simulink model "CAVE_MachE_Simulink_250904"  (R2024a)
settings: configuration reference "ConfigSetDesktopFixedStep" (kept outside this file)
PreLoadFcn:
  | VSS_BICYCLE=Simulink.Variant('Dual=0');
  | VSS_DUAL=Simulink.Variant('Dual=1');
  | Dual=1;
  | load('DriveCycle2.mat')
PostLoadFcn:
  | if any(exist('dsrtsu_mdlpostloadfcn', 'file') ~= 0), dsrtsu_mdlpostloadfcn('Execute', bdroot); end
InitFcn:
  | , if any(exist('rtifpga_mdlclblib', 'file') ~= 0), rtifpga_mdlclblib('Init', bdroot); end,
  | , if any(exist('dsmpb_private', 'file') ~= 0), dsmpb_private('dsmpb_mdlclblib', 'Init', bdroot); end,
  | load('DriveCycle2.mat')
model workspace (MAT data in the model file):
  Gas = 0.383333333333
values from neighbouring files (symbols this model uses):
  CoastDown =     [Run_Simulink.mat]
  limitedMCT =     [Run_Simulink.mat]
  MCT =     [Run_Simulink.mat]
  pMCT =     [Run_Simulink.mat]
  RealSimPara =     [Run_Simulink.mat]
  Ref_speed = [13 13.007895099 13.015778396 13.023649891 13.031509584 13.039357475 13.047193564 13.055017851 13.062830336 13.070631019 13.0784199 13.086196979 ... (2669 elements, 2669x1)]    [Ref_speed_and_time.mat]
  Ref_time = [0 0.01 0.02 0.03 0.04 0.05 0.06 0.07 0.08 0.09 0.1 0.11 ... (2669 elements, 2669x1)]    [Ref_speed_and_time.mat]
  US06 =     [Run_Simulink.mat]
undefined symbols (not defined in the file or in its folder): AccelCmd, ActTqLF_Nm_, ActTqLR_Nm_, ActTqRF_Nm_, ActTqRR_Nm_, BattChargeLimitMaxPwr, BattChargeLimitSocBpts, BattChargeLimitTbl, BattChrgCapcty, BattDischargeLimitSocBpts, BattDischargeLimitTbl, BattDischargeMaxPwr, BattNumCellsParallel, BattNumCellsSeries, BattOpenVoltCapBpts, BattOpenVoltTbl, BattResistSocBpts, BattResistTbl, BattResistTempBpts, BrakeMaxPrs, BrakeMaxTrq, ChassisDistCg2FrontAxle, ChassisDistCg2RearAxle, ChassisVehMass, CltchCmd, DecelCmd, DiffRatio, DiscIntNeverNeededParam, EnvGravCnst, EnvPrs, EnvTemp, FuelSpecificGrav, GearCmd, h, InitStates, lgSw, MtrEffSpdBpts, MtrEffTbl, MtrEffTrqBpts, MtrPwrMax, MtrTrqMax, SteeringCmd, SupvsryCtrlRegenBrkCutOffTbl, SupvsryCtrlRegenSpdBpts, TestScnrioCycleNum, VEH
libraries: VSIGenLib x122, simulink x108, etargetslib x75, dsmpblib x41, vehdynlibtire x24, autolibshared x19, vehdynlibsuspension x14, vehdynlibtirecommon x14, autolibutils x10, CarMaker4SL x8, VsrLibWheel x8, autolibpowerinfoutils x6
(part 4 of 29)

== system CAVE_MachE_Simulink_250904/Vehicle Under Test2/Vehicle/Motor ==
  SupvsryCtrl : Inport
  MtrSpd : Inport  Port=2
  Bus Creator1 : BusCreator  Inputs=1
  Bus Creator2 : BusCreator  Inputs=4
  Bus Selector1 : BusSelector  OutputSignals=Volt
  Bus Selector2 : BusSelector  OutputSignals=MtrTrqCmd
  Bus Selector3 : BusSelector  OutputSignals=PwrInfo.PwrTrnsfrd.PwrMtr,PwrInfo.PwrTrnsfrd.PwrBus
  Mach-E Motor : autolibmappedmotor/Mapped Motor  port_config=Speed  param_by=Maximum torque and power  w_t=[ 0 375 750 800 ]  T_t=[0.09 0.08 0.07 0]  torque_max=800  power_max=358000  Tc=0.01  param_loss=Tabulated efficiency data  eff=100  w_eff=375  T_eff=0.08  Piron=0  Pbase=0  w_eff_bp=MtrEffSpdBpts.*pi/30  T_eff_bp=MtrEffTrqBpts  Temp_eff_bp=[233.15 293.15 373.15]  losses_table=[1 2;3 4]  losses_table_3d=cat(3,[1.49 1.67 2.21 3.10; 0.42 0.69 1.14 2.03; 0.06 0.24 0.78 1.68; 0.42 0.69 1.14 2.03; 1.49 1.67 2.21 3.10],[1.49 1.67 2.21 3.10; 0.42 0.69 1.14 2.03; 0.06 0.24 0.78 1.68; 0.42 0.69 1.14 2.03; 1.49 1.67 2.21 3.10],[1.49 1.67 2.21 3.10; 0.42 0.69 1.14 2.03; 0.06 0.24 0.78 1.68; 0.42 0.69 1.14 2.03; 1.49 1.67 2.21 3.10])  efficiency_table=MtrEffTbl*0.94  efficiency_table_3d=cat(3,[95 95 95 95; 95 95 95 95; 95 95 95 95; 95 95 95 95; 95 95 95 95],[95 95 95 95; 95 95 95 95; 95 95 95 95; 95 95 95 95; 95 95 95 95],[95 95 95 95; 95 95 95 95; 95 95 95 95; 95 95 95 95; 95 95 95 95])  J=5e-6  b=1e-5  omega_o=0  T_t_extended=[0 0.07 0.08 0.09 0.08 0.07 0]  w_t_extended=[-800 -750 -375 0 375 750 800]  KLossIron=0  KLossCopper=0  x_w_eff_vec=[-1047.1975511966 -942.477796076938 -837.758040957278 -733.038285837618 -628.318530717959 -523.598775598299 -418.879020478639 -314.159265358979 -285.714285713875 -209.43951023932 -104.71975511966 0 104.71975511966 209.43951023932 285.714285713875 314.159265358979 418.879020478639 523.598775598299 628.318530717959 733.038285837618 837.758040957278 942.477796076938 1047.1975511966]  x_T_eff_vec=[-360 -334.285714285714 -308.571428571429 -282.857142857143 -257.142857142857 -231.428571428571 -205.714285714286 -180 -154.285714285714 -128.571428571429 -102.857142857143 -77.1428571428572 -51.4285714285714 -25.7142857142857 0 25.7142857142857 51.4285714285714 77.1428571428572 102.857142857143 128.571428571429 154.285714285714 180 205.714285714286 231.428571428571 257.142857142857 282.857142857143 308.571428571429 334.285714285714 360]  x_tmp_eff_vec=[-0.09 -0.06 -0.03 0 0.03 0.06 0.09]  x_losses_mat=[54250.1517943165 50375.1409518653 46500.1301094142 42625.119266963 38750.1084245118 34875.0975820605 31000.0867396095 27125.0758971582 23250.065054707 19375.054212256 15500.0433698047 12629.4764797412 9803.55154311708 6774.11181875432 0 5412.5153431847 8293.80460547705 10921.9712596802 13550.1379138833 16937.6723923542 20325.2068708249 23712.7413492957 27100.2758277666 30487.8103062373 33875.3447847082 37262.879263179 40650.4137416499 44037.9482201206 47425.4826985915;44696.230836134 41503.6429192672 38311.0550024006 35118.4670855338 31925.8791686671 28733.2912518003 25540.7033349337 22348.115418067 19155.5275012002 15962.9395843336 12770.3516674669 9577.76375060014 6975.01951641212 6096.70063687888 0 4871.26380886623 6097.56206124747 8462.91205003029 11283.8827333737 14104.8534167172 16925.8241000605 19746.794783404 22567.7654667475 25388.7361500908 28209.7068334343 31030.6775167777 33851.6482001212 36672.6188834645 39493.589566808;36137.1105685043 33555.8883850397 30974.6662015752 28393.4440181105 25812.2218346459 23230.9996511813 20649.7774677168 18068.5552842522 15487.3331007875 12906.110917323 10324.8887338584 8513.56777831124 6200.01734792188 5419.28945500345 0 4330.01227454776 5420.05516555331 7522.58848891581 9220.12563933554 11525.1570491694 13830.1884590033 16135.2198688372 18440.2512786711 20745.2826885049 23050.3140983388 25355.3455081727 27660.3769180066 29965.4083278404 32270.4397376744;31619.9717474413 29361.4023369097 27102.8329263783 24844.2635158467 22585.6941053152 20327.1246947836 18068.5552842522 15809.9858737206 13551.4164631891 11292.8470526576 9034.27764212609 7449.37180602233 5425.01517943165 4741.87827312802 0 3788.76074022929 4742.54826985915 6582.26492780134 8067.6099344186 10084.5124180233 12101.4149016279 14118.3173852325 16135.2198688372 18152.1223524418 20169.0248360465 22185.9273196511 24202.8298032558 26219.7322868604 28236.6347704651;27102.8329263782 25166.9162887798 23230.9996511814 21295.0830135829 19359.1663759844 17423.249738386 15487.3331007876 13551.4164631891 11615.4998255906 9679.58318799226 8513.56777831124 6385.17583373343 4650.01301094141 4064.46709125259 0 3247.50920591082 4065.04137416498 5641.94136668686 7522.58848891582 8643.86778687709 10372.6413442524 12101.4149016279 13830.1884590033 15558.9620163787 17287.7355737541 19016.5091311295 20745.282688505 22474.0562458803 24202.8298032558;22585.6941053152 20972.4302406498 19359.1663759845 17745.9025113191 16132.6386466537 14519.3747819883 12906.110917323 11292.8470526576 9679.58318799221 8066.31932332688 7094.63981525937 5320.97986144452 3875.01084245118 3387.05590937716 0 2706.25767159235 3387.53447847082 4701.61780557238 6268.82374076318 7203.22315573091 8643.86778687704 10084.5124180232 11525.1570491694 12965.8016803156 14406.4463114618 15847.0909426079 17287.7355737541 18728.3802049003 20169.0248360465;19864.9914827262 18446.0635196743 17027.1355566225 15608.2075935706 14189.2796305187 12770.3516674668 11351.423704415 9932.4957413631 8513.56777831121 7094.63981525938 5675.71185220749 4256.78388915562 3100.00867396094 2709.64472750173 0 2165.00613727388 2710.02758277665 3761.29424445791 5015.05899261055 6268.82374076319 7522.58848891579 8776.35323706844 10030.1179852211 11283.8827333737 12537.6474815263 13791.412229679 15045.1769778316 16298.9417259842 17552.7064741369;20587.4582405459 19116.9255090783 17646.3927776108 16175.8600461432 12629.4764797412 11366.528831767 10103.581183793 8137.52276914747 6975.01951641211 5812.51626367679 4650.01301094142 3788.84294392236 2525.89529594824 2032.23354562629 0 1623.75460295541 2184.39425193603 3276.59137790406 4065.04137416499 5081.30171770625 6097.56206124746 7113.82240478872 8737.57700774416 9829.77413371214 10921.9712596802 13684.7775990372 14928.8482898587 16172.9189806802 17416.9896715018;18723.4042552922 17386.0182370571 16048.6322188219 14711.2462005868 11485.9634880614 10337.3671392553 9188.77079044916 8040.174441643 6891.57809283685 5742.98174403074 4594.38539522458 ...(+6536 chars)]  x_losses_mat_3d=[37.8947368421052 25.2631578947368 12.6315789473684 0 12 24 36;18.9473684210526 12.6315789473684 6.3157894736842 0 5.99999999999999 12 18;0 0 0 0 0 0 0;18 12 5.99999999999999 0 6.3157894736842 12.6315789473684 18.9473684210526;36 24 12 0 12.6315789473684 25.2631578947368 37.8947368421052]  CalLossMapData={}  CalLossWithTempMapData={}  aMode=aMode  RefBlkName='autolibmappedmotor/Mapped Motor'
  Mapped Motor : autolibmappedmotor/Mapped Motor  port_config=Speed  param_by=Maximum torque and power  w_t=[ 0 375 750 800 ]  T_t=[0.09 0.08 0.07 0]  torque_max=MtrTrqMax  power_max=MtrPwrMax  Tc=MtrTrqTimeCnst  param_loss=Tabulated efficiency data  eff=100  w_eff=375  T_eff=0.08  Piron=0  Pbase=0  w_eff_bp=MtrEffSpdBpts.*pi/30  T_eff_bp=MtrEffTrqBpts  Temp_eff_bp=[233.15 293.15 373.15]  losses_table=[1 2;3 4]  losses_table_3d=cat(3,[1.49 1.67 2.21 3.10; 0.42 0.69 1.14 2.03; 0.06 0.24 0.78 1.68; 0.42 0.69 1.14 2.03; 1.49 1.67 2.21 3.10],[1.49 1.67 2.21 3.10; 0.42 0.69 1.14 2.03; 0.06 0.24 0.78 1.68; 0.42 0.69 1.14 2.03; 1.49 1.67 2.21 3.10],[1.49 1.67 2.21 3.10; 0.42 0.69 1.14 2.03; 0.06 0.24 0.78 1.68; 0.42 0.69 1.14 2.03; 1.49 1.67 2.21 3.10])  efficiency_table=MtrEffTbl*0.94  efficiency_table_3d=cat(3,[95 95 95 95; 95 95 95 95; 95 95 95 95; 95 95 95 95; 95 95 95 95],[95 95 95 95; 95 95 95 95; 95 95 95 95; 95 95 95 95; 95 95 95 95],[95 95 95 95; 95 95 95 95; 95 95 95 95; 95 95 95 95; 95 95 95 95])  J=5e-6  b=1e-5  omega_o=0  T_t_extended=[0 0.07 0.08 0.09 0.08 0.07 0]  w_t_extended=[-800 -750 -375 0 375 750 800]  KLossIron=0  KLossCopper=0  x_w_eff_vec=[-1047.1975511966 -942.477796076938 -837.758040957278 -733.038285837618 -628.318530717959 -523.598775598299 -418.879020478639 -314.159265358979 -285.714285713875 -209.43951023932 -104.71975511966 0 104.71975511966 209.43951023932 285.714285713875 314.159265358979 418.879020478639 523.598775598299 628.318530717959 733.038285837618 837.758040957278 942.477796076938 1047.1975511966]  x_T_eff_vec=[-360 -334.285714285714 -308.571428571429 -282.857142857143 -257.142857142857 -231.428571428571 -205.714285714286 -180 -154.285714285714 -128.571428571429 -102.857142857143 -77.1428571428572 -51.4285714285714 -25.7142857142857 0 25.7142857142857 51.4285714285714 77.1428571428572 102.857142857143 128.571428571429 154.285714285714 180 205.714285714286 231.428571428571 257.142857142857 282.857142857143 308.571428571429 334.285714285714 360]  x_tmp_eff_vec=[-0.09 -0.06 -0.03 0 0.03 0.06 0.09]  x_losses_mat=[54250.1517943165 50375.1409518653 46500.1301094142 42625.119266963 38750.1084245118 34875.0975820605 31000.0867396095 27125.0758971582 23250.065054707 19375.054212256 15500.0433698047 12629.4764797412 9803.55154311708 6774.11181875432 0 5412.5153431847 8293.80460547705 10921.9712596802 13550.1379138833 16937.6723923542 20325.2068708249 23712.7413492957 27100.2758277666 30487.8103062373 33875.3447847082 37262.879263179 40650.4137416499 44037.9482201206 47425.4826985915;44696.230836134 41503.6429192672 38311.0550024006 35118.4670855338 31925.8791686671 28733.2912518003 25540.7033349337 22348.115418067 19155.5275012002 15962.9395843336 12770.3516674669 9577.76375060014 6975.01951641212 6096.70063687888 0 4871.26380886623 6097.56206124747 8462.91205003029 11283.8827333737 14104.8534167172 16925.8241000605 19746.794783404 22567.7654667475 25388.7361500908 28209.7068334343 31030.6775167777 33851.6482001212 36672.6188834645 39493.589566808;36137.1105685043 33555.8883850397 30974.6662015752 28393.4440181105 25812.2218346459 23230.9996511813 20649.7774677168 18068.5552842522 15487.3331007875 12906.110917323 10324.8887338584 8513.56777831124 6200.01734792188 5419.28945500345 0 4330.01227454776 5420.05516555331 7522.58848891581 9220.12563933554 11525.1570491694 13830.1884590033 16135.2198688372 18440.2512786711 20745.2826885049 23050.3140983388 25355.3455081727 27660.3769180066 29965.4083278404 32270.4397376744;31619.9717474413 29361.4023369097 27102.8329263783 24844.2635158467 22585.6941053152 20327.1246947836 18068.5552842522 15809.9858737206 13551.4164631891 11292.8470526576 9034.27764212609 7449.37180602233 5425.01517943165 4741.87827312802 0 3788.76074022929 4742.54826985915 6582.26492780134 8067.6099344186 10084.5124180233 12101.4149016279 14118.3173852325 16135.2198688372 18152.1223524418 20169.0248360465 22185.9273196511 24202.8298032558 26219.7322868604 28236.6347704651;27102.8329263782 25166.9162887798 23230.9996511814 21295.0830135829 19359.1663759844 17423.249738386 15487.3331007876 13551.4164631891 11615.4998255906 9679.58318799226 8513.56777831124 6385.17583373343 4650.01301094141 4064.46709125259 0 3247.50920591082 4065.04137416498 5641.94136668686 7522.58848891582 8643.86778687709 10372.6413442524 12101.4149016279 13830.1884590033 15558.9620163787 17287.7355737541 19016.5091311295 20745.282688505 22474.0562458803 24202.8298032558;22585.6941053152 20972.4302406498 19359.1663759845 17745.9025113191 16132.6386466537 14519.3747819883 12906.110917323 11292.8470526576 9679.58318799221 8066.31932332688 7094.63981525937 5320.97986144452 3875.01084245118 3387.05590937716 0 2706.25767159235 3387.53447847082 4701.61780557238 6268.82374076318 7203.22315573091 8643.86778687704 10084.5124180232 11525.1570491694 12965.8016803156 14406.4463114618 15847.0909426079 17287.7355737541 18728.3802049003 20169.0248360465;19864.9914827262 18446.0635196743 17027.1355566225 15608.2075935706 14189.2796305187 12770.3516674668 11351.423704415 9932.4957413631 8513.56777831121 7094.63981525938 5675.71185220749 4256.78388915562 3100.00867396094 2709.64472750173 0 2165.00613727388 2710.02758277665 3761.29424445791 5015.05899261055 6268.82374076319 7522.58848891579 8776.35323706844 10030.1179852211 11283.8827333737 12537.6474815263 13791.412229679 15045.1769778316 16298.9417259842 17552.7064741369;20587.4582405459 19116.9255090783 17646.3927776108 16175.8600461432 12629.4764797412 11366.528831767 10103.581183793 8137.52276914747 6975.01951641211 5812.51626367679 4650.01301094142 3788.84294392236 2525.89529594824 2032.23354562629 0 1623.75460295541 2184.39425193603 3276.59137790406 4065.04137416499 5081.30171770625 6097.56206124746 7113.82240478872 8737.57700774416 9829.77413371214 10921.9712596802 13684.7775990372 14928.8482898587 16172.9189806802 17416.9896715018;18723.4042552922 17386.0182370571 16048.6322188219 14711.2462005868 11485.9634880614 10337.3671392553 9188.77079044916 8040.174441643 6891.57809283685 5742.98174403074 4594.38539522458 ...(+6536 chars)]  x_losses_mat_3d=[37.8947368421052 25.2631578947368 12.6315789473684 0 12 24 36;18.9473684210526 12.6315789473684 6.3157894736842 0 5.99999999999999 12 18;0 0 0 0 0 0 0;18 12 5.99999999999999 0 6.3157894736842 12.6315789473684 18.9473684210526;36 24 12 0 12.6315789473684 25.2631578947368 37.8947368421052]  CalLossMapData={}  CalLossWithTempMapData={}  aMode=aMode  RefBlkName='autolibmappedmotor/Mapped Motor'
  Memory : Memory
  Mux{,1..3} (4 alike) : Mux  Inputs=1
  Two-Way Connection1 : TwoWayConnection
  Batt : PMIOPort  Side=Left
  Mtr : Outport
  MtrTrq : Outport  Port=2
  wires:
  Mach-E Motor/3 -> Mux/1, MtrTrq/1  "Trq"
  Mach-E Motor/2 -> Memory/1  "Curr"
  Bus Creator1/1 -> Two-Way Connection1/1
  Mach-E Motor/1 -> Bus Selector3/1
  SupvsryCtrl/1 -> Bus Selector2/1
  Two-Way Connection1/1 -> Bus Selector1/1
  Bus Selector1/1 -> Mach-E Motor/1  "<Volt>"
  Bus Selector2/1 -> Mach-E Motor/3  "<MtrTrqCmd>"
  Mux/1 -> Bus Creator2/2  "MtrTrq"
  Bus Creator2/1 -> Mtr/1
  Mux2/1 -> Bus Creator2/3  "MtrMechPwr"
  Bus Selector3/1 -> Mux2/1  "<PwrMtr>"
  Mux1/1 -> Bus Creator2/1  "MtrSpd"
  Bus Selector3/2 -> Mux3/1  "<PwrBus>"
  Mux3/1 -> Bus Creator2/4  "MtrElecPwr"
  Memory/1 -> Bus Creator1/1  "Curr"
  MtrSpd/1 -> Mach-E Motor/2, Mux1/1
  connections:
  Batt/RConn1 -- Two-Way Connection1/RConn1

== system CAVE_MachE_Simulink_250904/Vehicle Under Test2/Vehicle/Powertrain Supervisory Controller  ==
  Driver : Inport
  Chassis : Inport  Port=2
  Mtr : Inport  Port=3
  Batt : Inport  Port=4
  Bus Selector : BusSelector  OutputSignals=SteeringCmd
  Engine Torque Command : Subsystem
  Scope : Scope  NumInputPorts=4
  Subsystem1 : Subsystem
      mask Display: disp('')
  Subsystem4 : Subsystem
      mask Display: disp('')
  SupvsryCtrl : Outport
  wires:
  Engine Torque Command/4(DriverGearCmd) -> Scope/4, Subsystem1/4(DriverGearCmd)  "DriverGearCmd"
  Engine Torque Command/3(BrkCmd) -> Scope/3, Subsystem1/3(BrkCmd)  "BrkCmd"
  Engine Torque Command/2(AccelCmd) -> Scope/2, Subsystem1/2(AccelCmd)  "AccelCmd"
  Engine Torque Command/1(MtrTrqCmd) -> Scope/1, Subsystem1/1(MtrTrqCmd)  "MtrTrqCmd"
  Subsystem4/6(MtrSpd) -> Engine Torque Command/6(MtrSpd)
  Subsystem4/5(BattSoc) -> Engine Torque Command/5(BattSoc)
  Subsystem4/4(VehSpd) -> Engine Torque Command/4(VehSpd)
  Subsystem4/3(DriverGearCmd) -> Engine Torque Command/3(DriverGearCmdIn)
  Mtr/1 -> Subsystem4/4(Mtr)
  Subsystem1/1(SupvsryCtrl) -> SupvsryCtrl/1
  Batt/1 -> Subsystem4/3(Batt)
  Chassis/1 -> Subsystem4/2(Chassis)
  Driver/1 -> Bus Selector/1, Subsystem4/1(Driver)
  Subsystem4/1(AccelCmd) -> Engine Torque Command/1(AccelCmdIn)
  Subsystem4/2(DecelCmd) -> Engine Torque Command/2(DecelCmdIn)
  Bus Selector/1 -> Subsystem1/5(SteeringCmd)  "<SteeringCmd>"

== system CAVE_MachE_Simulink_250904/Vehicle Under Test2/Vehicle/Rototest UDP RX ExternalMode   ==
  RotoTest ExternalControlEthernet : dsmpblib/Data Inport  Priority=10000
      settings: SourceProductName=dSPACE Model Interface Package for Simulink (MIPS)
  Terminator{1..5,10..11} (7 alike) : Terminator
  UDP Receive (1) : dsmpblib/Data Inport  Priority=10000
      settings: SourceProductName=dSPACE Model Interface Package for Simulink (MIPS)
  UDP Transmit (4)_In : dsmpblib/Data Inport  Priority=10000
      settings: SourceProductName=dSPACE Model Interface Package for Simulink (MIPS)
  Data Vector : Outport
  wires:
  UDP Receive (1)/4 -> Terminator4/1
  UDP Receive (1)/3 -> Terminator3/1
  UDP Transmit (4)_In/1 -> Terminator10/1
  UDP Receive (1)/5 -> Terminator5/1
  UDP Receive (1)/2 -> Terminator2/1
  UDP Transmit (4)_In/2 -> Terminator11/1
  UDP Receive (1)/1 -> Data Vector/1
  RotoTest ExternalControlEthernet/1 -> Terminator1/1

== system CAVE_MachE_Simulink_250904/Vehicle Under Test2/Vehicle/Rototest UDP TX ExternalMode   ==
  Rototest_UDP_TX : Inport
  UDP Transmit (4)_Out : dsmpblib/Data Outport  Priority=-10000
      settings: SourceProductName=dSPACE Model Interface Package for Simulink (MIPS)
  wires:
  Rototest_UDP_TX/1 -> UDP Transmit (4)_Out/1

== system CAVE_MachE_Simulink_250904/Vehicle Under Test2/Vehicle/Rototest and ORNL Interface ==
  note: rad/s
  CarTrqT2W : Inport
  UDP Input : Inport  Port=2
  BRAKE_PRESSED : Inport  Port=3
  vehSpeedKph : Inport  Port=4
  FXIN : Inport  Port=5
  1/tireRadius : Gain  Gain=1/0.3232
  ChargingMode : Constant  Value=0
  CmdSpeed (mph) : Constant  Value=0
  Constant : Constant  Value=3000
  DriverSwitch : Constant  Value=0
  DummyPT : Subsystem
  Format CM Powertrain Signals : Subsystem
  From Rototest : Subsystem
  Get Wheel Spd Cmd Based on Wheel Dynamics : Subsystem
  Multiport Switch : MultiPortSwitch  DataPortOrder=Zero-based contiguous  Inputs=2  zeroidx=on  SaturateOnIntegerOverflow=off  InputSameDT=off
  Multiport Switch1 : MultiPortSwitch  DataPortOrder=Zero-based contiguous  Inputs=2  zeroidx=on  SaturateOnIntegerOverflow=off  InputSameDT=off
  RotoTrqPreprocess : Subsystem
  Scope : Scope
  Scope1 : Scope
  Subsystem2 : Subsystem
  Terminator2 : Terminator
  To Rototest with Band-Aid : Subsystem
  mph2m/s : Gain  Gain=0.44704
  BrakeUpd : Outport
  Powertrain Out : Outport  Port=2
  DataSend : Outport  Port=3
  WhlSpd : Outport  Port=4
  wires:
  [MaxRegen] -> Get Wheel Spd Cmd Based on Wheel Dynamics/4(MaxRegen)
  [MaxRegen] -> Format CM Powertrain Signals/4(MaxRegen)
  Get Wheel Spd Cmd Based on Wheel Dynamics/1(WhlSpdCmd) -> WhlSpd/1, To Rototest with Band-Aid/1(SpeedCmd_rps), Scope1/1, DummyPT/1(WhlSpeedIn), Multiport Switch1/2  "WhlSpdCmd"
  Multiport Switch/1 -> Scope/1, Get Wheel Spd Cmd Based on Wheel Dynamics/3(AxlTrq)
  RotoTrqPreprocess/2(AxleTrqVeh) -> Format CM Powertrain Signals/3(AxlTrq), Multiport Switch/2
  [AxlTrqRoto] -> To Rototest with Band-Aid/2(AxleTrq_roto_Nm)
  Format CM Powertrain Signals/1(PowerTrainOutIdeal) -> Powertrain Out/1
  DriverSwitch/1 -> Multiport Switch/1
  Subsystem2/1(BrakeUpd) -> BrakeUpd/1, Get Wheel Spd Cmd Based on Wheel Dynamics/1(BrakingTorques), Format CM Powertrain Signals/1(BrakingTorques)
  CarTrqT2W/1 -> Get Wheel Spd Cmd Based on Wheel Dynamics/2(Trq_T2W)
  DummyPT/1(WheelTorqueOut) -> Multiport Switch/3
  To Rototest with Band-Aid/1(Out1) -> DataSend/1  "DataSend"
  Constant/1 -> [MaxRegen]
  BRAKE_PRESSED/1 -> To Rototest with Band-Aid/3(BRAKE_PRESSED)
  Multiport Switch1/1 -> Format CM Powertrain Signals/2(RotoWheelSpd)
  ChargingMode/1 -> Multiport Switch1/1
  CmdSpeed (mph)/1 -> mph2m/s/1
  1/tireRadius/1 -> Multiport Switch1/3
  mph2m/s/1 -> 1/tireRadius/1
  FXIN/1 -> Get Wheel Spd Cmd Based on Wheel Dynamics/5(FxIn)
  UDP Input/1 -> From Rototest/1(Input)
  From Rototest/1(SpdAct) -> Terminator2/1
  From Rototest/2(AxlTrq) -> Subsystem2/1(AxlTorq), RotoTrqPreprocess/1(AxleTrqRaw)
  vehSpeedKph/1 -> To Rototest with Band-Aid/4(Vehicle_Speed_kph)  "vehSpeedKph"
  RotoTrqPreprocess/1(AxleTrqRoto) -> [AxlTrqRoto]

== system CAVE_MachE_Simulink_250904/Vehicle Under Test2/Vehicle/Vehicle Dynamics ==
  Env : Inport
  SupvsryCtrl : Inport  Port=2
  AxlTrq : Inport  Port=3
  Vehicle 14DOF : Subsystem  VariantControl=Veh14DOF
  Vehicle 7DOF : Subsystem  VariantControl=Veh7DOF
  Vehicle Longitudinal : Subsystem  VariantControl=VehLong
  Whl : Outport
  Chassis : Outport  Port=2
  RototestInput : Outport  Port=3

== system CAVE_MachE_Simulink_250904/Vehicle Under Test3/Environment/Ground Feedback ==
  note: 1) Add Subsystem or Model blocks as valid variant choices.
      | 2) You cannot connect blocks at this level. At simulation, connectivity is automatically
      | determined, based on the active variant and port name matching.
  Friction : Inport
  Ground Z Level : Inport  Port=2
  3D Engine : Subsystem  VariantControl=1
  Constant : Subsystem  VariantControl=0
  Ground : Outport  VectorParamsAs1DForOutWhenUnconnected=off

== system CAVE_MachE_Simulink_250904/Vehicle Under Test3/Environment/Subsystem ==
  Grade : Inport
  Constant : Constant  Value=EnvPrs
  Constant1 : Constant  Value=EnvTemp
  Constant2 : Constant  Value=0
  Constant3 : Constant  Value=0
  Constant4 : Constant  Value=0
  Signal Specification : SignalSpecification  Unit=Pa
  Signal Specification1 : SignalSpecification  Unit=K
  Signal Specification2 : SignalSpecification  Unit=rad
  Signal Specification3 : SignalSpecification  Unit=m/s
  Signal Specification4 : SignalSpecification  Unit=m/s
  Signal Specification5 : SignalSpecification  Unit=m/s
  Vector Concatenate : Concatenate  NumInputs=3
  EnvPrs : Outport
  EnvTemp : Outport  Port=2
  WindVel : Outport  Port=3
  RoadGrade : Outport  Port=4
  wires:
  Constant/1 -> Signal Specification/1
  Constant2/1 -> Signal Specification3/1
  Constant1/1 -> Signal Specification1/1
  Grade/1 -> Signal Specification2/1
  Signal Specification/1 -> EnvPrs/1
  Signal Specification1/1 -> EnvTemp/1
  Signal Specification2/1 -> RoadGrade/1
  Vector Concatenate/1 -> WindVel/1
  Signal Specification3/1 -> Vector Concatenate/1  "WindX"
  Constant3/1 -> Signal Specification4/1
  Constant4/1 -> Signal Specification5/1
  Signal Specification4/1 -> Vector Concatenate/2  "WindY"
  Signal Specification5/1 -> Vector Concatenate/3  "WindZ"

== system CAVE_MachE_Simulink_250904/Vehicle Under Test3/Environment/Subsystem1 ==
  EnvPrs : Inport
  EnvTemp : Inport  Port=2
  WindVel : Inport  Port=3
  RoadGrade : Inport  Port=4
  GroundBus : Inport  Port=5
  Bus Creator : BusCreator  Inputs=5
  Env : Outport
  wires:
  EnvPrs/1 -> Bus Creator/1  "EnvPrs"
  EnvTemp/1 -> Bus Creator/2  "EnvTemp"
  Bus Creator/1 -> Env/1  "Env"
  WindVel/1 -> Bus Creator/3  "WindVel"
  RoadGrade/1 -> Bus Creator/4  "RoadGrade"
  GroundBus/1 -> Bus Creator/5  "GndBus"

== system CAVE_MachE_Simulink_250904/Vehicle Under Test3/Monitor/Calculate Fuel MPG ==
  Monitor : Inport
  Bus Selector : BusSelector  OutputSignals=Veh.Chassis.VehDist,Veh.Batt.EngPlant.FuellMassFlw
  Constant : Constant  Value=FuelSpecificGrav
  Density of Water : Gain  Gain=997
  Divide : Product  Inputs=*/
  Divide1 : Product  Inputs=*/
  Integrator : Integrator
  Saturation : Saturate  UpperLimit=inf  LowerLimit=1e-7
  Signal Specification : SignalSpecification  Unit=mi
  Signal Specification1 : SignalSpecification  Unit=m^3
  Signal Specification2 : SignalSpecification  Unit=gal
  Unit Conversion : UnitConversion
  Unit Conversion1 : UnitConversion
  FuelEconMPG : Outport
  wires:
  Divide1/1 -> FuelEconMPG/1  "FuelEconMPG"
  Divide/1 -> Signal Specification1/1
  Unit Conversion1/1 -> Signal Specification2/1
  Signal Specification2/1 -> Saturation/1
  Unit Conversion/1 -> Signal Specification/1
  Bus Selector/1 -> Unit Conversion/1  "<VehDist>"
  Bus Selector/2 -> Integrator/1  "<FuellMassFlw>"
  Integrator/1 -> Divide/1  "FuelMass"
  Density of Water/1 -> Divide/2
  Saturation/1 -> Divide1/2  "FuelVolume"
  Constant/1 -> Density of Water/1
  Signal Specification1/1 -> Unit Conversion1/1
  Monitor/1 -> Bus Selector/1
  Signal Specification/1 -> Divide1/1  "VehDistMiles"

== system CAVE_MachE_Simulink_250904/Vehicle Under Test3/Monitor/Calculate Powertrain Energy ==
  Monitor : Inport
  Bus Selector2 : BusSelector  OutputSignals=Veh.Diff.PwrInfo.PwrTrnsfrd.PwrTrnsfrd.PwrDriveshft
  Integrator : Integrator
  Signal Specification : SignalSpecification  Unit=J
  Signal Specification1 : SignalSpecification  Unit=kW*h
  Unit Conversion : UnitConversion
  TransEnrgyOutkWh : Outport
  wires:
  Unit Conversion/1 -> Signal Specification1/1
  Integrator/1 -> Signal Specification/1  "EnrgyTrans"
  Signal Specification/1 -> Unit Conversion/1
  Signal Specification1/1 -> TransEnrgyOutkWh/1
  Monitor/1 -> Bus Selector2/1
  Bus Selector2/1 -> Integrator/1  "<PwrDriveshft>"

== system CAVE_MachE_Simulink_250904/Vehicle Under Test3/Vehicle/Actuation and Outputs ==
  note: Driver Commands are [0,100] for both pedal and brake
  Driver Commands : Inport
  CarlaGBS : Inport  Port=2
  APP : Constant  Value=0
  AR_limit : Saturate  UpperLimit=65  LowerLimit=0
  BR_command_0to100 : Constant  Value=0
  BR_limit : Saturate  UpperLimit=70  LowerLimit=0
  Bus Creator : BusCreator  Inputs=2
  Bus Selector1 : BusSelector  OutputSignals=AccelPedalCmd
  Bus Selector3 : BusSelector  OutputSignals=BrakePedalCmd
  Constant : Constant  Value=0
  Constant1 : Constant  Value=0
  Demux : Demux  Outputs=3
  Gain : Gain  Gain=100
  Gain1 : Gain  Gain=100
  MOOG Brake Actuator : Subsystem
  Min threshold for Brake switch : Constant  Value=0
  Multiport Switch1 : MultiPortSwitch  Inputs=4  SaturateOnIntegerOverflow=off  InputSameDT=off
  Multiport Switch2 : MultiPortSwitch  Inputs=4  SaturateOnIntegerOverflow=off  InputSameDT=off
  Pedal Robot Control Selection : Constant  Value=2
  Relational Operator : RelationalOperator  Operator=>  OutDataTypeStr=boolean  InputSameDT=off
  Scope1 : Scope  NumInputPorts=2
  Vehicle Accel Pedal Voltage Output : Subsystem
  bped2br_N : Lookup_n-D  NumberOfTableDimensions=1  BreakpointsForDimension1=[0 0.1 0.2 100]  Table=[0 0 25 100]  InternalRulePriority=Speed  RndMeth=Simplest
  BrakeSwitch : Outport  VectorParamsAs1DForOutWhenUnconnected=off
  CAVE_Driver : Outport  Port=2
  tag scope: BrakeDriver=global, CarlaSteer=global, GasDriver=global
  wires:
  Multiport Switch1/1 -> AR_limit/1
  APP/1 -> Multiport Switch1/2
  Bus Selector1/1 -> Multiport Switch1/3  "<AccelPedalCmd>"
  Multiport Switch2/1 -> BR_limit/1
  Driver Commands/1 -> Bus Selector3/1, Bus Selector1/1
  Pedal Robot Control Selection/1 -> Multiport Switch1/1, Multiport Switch2/1
  BR_command_0to100/1 -> Multiport Switch2/2
  Bus Selector3/1 -> Multiport Switch2/3  "<BrakePedalCmd>"
  bped2br_N/1 -> MOOG Brake Actuator/1(Brake Pedal command [%])
  Min threshold for Brake switch/1 -> Relational Operator/2
  Relational Operator/1 -> BrakeSwitch/1  "BrakeSwitch"
  Constant/1 -> Multiport Switch1/5
  Constant1/1 -> Multiport Switch2/5
  Bus Creator/1 -> CAVE_Driver/1
  AR_limit/1 -> [GasDriver], Bus Creator/1, Vehicle Accel Pedal Voltage Output/1(APP_pct)  "AccelPedalCmd_pct"
  BR_limit/1 -> Bus Creator/2, [BrakeDriver], Relational Operator/1, bped2br_N/1  "BrakePedalCmd_pct"
  Demux/1 -> Gain/1
  Demux/2 -> Gain1/1
  CarlaGBS/1 -> Demux/1
  Gain/1 -> Multiport Switch1/4
  Gain1/1 -> Multiport Switch2/4
  Demux/3 -> [CarlaSteer]
  [GasDriver] -> Scope1/1
  [BrakeDriver] -> Scope1/2

== system CAVE_MachE_Simulink_250904/Vehicle Under Test3/Vehicle/Battery ==
  Battery : Subsystem
  Subsystem1 : Subsystem
      mask Display: disp('')
  BattOut : PMIOPort  Side=Right
  Batt : Outport
  wires:
  Battery/1(BattSoc) -> Subsystem1/1(BattSoc)
  Battery/2(BattCurr) -> Subsystem1/2(BattCurr)
  Battery/3(BattVolt) -> Subsystem1/3(BattVolt)
  Subsystem1/1(Batt) -> Batt/1
  connections:
  BattOut/RConn1 -- Battery/RConn1

== system CAVE_MachE_Simulink_250904/Vehicle Under Test3/Vehicle/Driver and Drive Cycle ==
  Veh speed feedback [kph] : Inport
  Veh speed cycle trigger : Inport  Port=2
  SUMO Veh speed Cmd Level : Inport  Port=3
  CarlaRef : Inport  Port=4
  1-D Lookup Table : Lookup_n-D  NumberOfTableDimensions=1  BreakpointsForDimension1=Ref_time  Table=Ref_speed  InternalRulePriority=Speed  RndMeth=Simplest
  Add : Sum
  Add1 : Sum  Inputs=+-
  Add2 : Sum
  Clock : Clock
  Clock1 : Clock
  CoastDown : Lookup_n-D  Commented=on  NumberOfTableDimensions=1  BreakpointsForDimension1=CoastDown.Time  Table=CoastDown.Speed  InternalRulePriority=Speed  RndMeth=Simplest
  Constant : Constant  Value=0
  Data Type Conversion11 : DataTypeConversion  OutDataTypeStr=double  SaturateOnIntegerOverflow=off  RndMeth=Floor  LockScale=on
  Demux : Demux  Outputs=3
  DriveCycleSelect : Constant  Commented=on
  Driver and PI with FF Control : Subsystem
  Gain : Gain  Gain=1/1.609
  Gain1 : Gain  Gain=1/1.609
  Gain2 : Gain  Gain=3.6
  Gain3 : Gain  Gain=3.6
  Get Cycle Clock Time : Subsystem
  MCT : Lookup_n-D  Commented=on  NumberOfTableDimensions=1  BreakpointsForDimension1=MCT.Time  Table=MCT.Speed  InternalRulePriority=Speed  RndMeth=Simplest
  ManSpd : Constant  Value=0
  ManSpdSel : Constant  Value=2
  Memory4 : Memory
  Multiport Switch : MultiPortSwitch  Commented=on  Inputs=5  SaturateOnIntegerOverflow=off  InputSameDT=off
  Multiport Switch1 : MultiPortSwitch  Inputs=4  SaturateOnIntegerOverflow=off  InputSameDT=off
  Rate Limiter : RateLimiter  RisingSlewLimit=5  FallingSlewLimit=-5  SampleTimeMode=inherited
  Scope : Scope  NumInputPorts=2
  Switch1 : Switch  Threshold=3  SaturateOnIntegerOverflow=off  InputSameDT=off
  Terminator{,1..3} (4 alike) : Terminator
  Terminator4 : Terminator  Commented=on
  US06 : Lookup_n-D  Commented=on  NumberOfTableDimensions=1  BreakpointsForDimension1=US06.Time  Table=US06.Speed  InternalRulePriority=Speed  RndMeth=Simplest
  US1 : Lookup_n-D  NumberOfTableDimensions=1  BreakpointsForDimension1=US06.Time  Table=US06.Speed  InternalRulePriority=Speed  RndMeth=Simplest
  driver look ahead seconds : Constant  Value=0.5
  limitedMCT : Lookup_n-D  Commented=on  NumberOfTableDimensions=1  BreakpointsForDimension1=limitedMCT.Time  Table=limitedMCT.Speed  InternalRulePriority=Speed  RndMeth=Simplest
  pMCT : Lookup_n-D  Commented=on  NumberOfTableDimensions=1  BreakpointsForDimension1=pMCT.Time  Table=pMCT.Speed  InternalRulePriority=Speed  RndMeth=Simplest
  DriverBus : Outport
  Output : Outport  Port=2
  wires:
  Veh speed cycle trigger/1 -> Get Cycle Clock Time/1(Cycle Trigger)
  MCT/1 -> Multiport Switch/5
  US06/1 -> Multiport Switch/4
  Add/1 -> CoastDown/1, pMCT/1, limitedMCT/1, MCT/1, US06/1
  CoastDown/1 -> Multiport Switch/2
  pMCT/1 -> Multiport Switch/3
  DriveCycleSelect/1 -> Multiport Switch/1
  [VehSpdKph] -> Data Type Conversion11/1
  Driver and PI with FF Control/1(DriverBus) -> DriverBus/1
  Data Type Conversion11/1 -> Gain/1, Scope/1, Driver and PI with FF Control/1(Vehicle_Spd_kph)  "Vehicle_Spd_kph"
  Get Cycle Clock Time/1(tCycle) -> Add/2
  driver look ahead seconds/1 -> Add/1
  limitedMCT/1 -> Multiport Switch/6
  Veh speed feedback [kph]/1 -> [VehSpdKph]
  Gain/1 -> Terminator/1  "Vehicle_Spd_mph"
  Gain1/1 -> Terminator1/1  "Vehicle_SpdDmd_mph"
  Multiport Switch1/1 -> Scope/2, Gain1/1, Driver and PI with FF Control/2(Vehicle_SpdDmd_kph)  "RefSpd [km/hr]"
  Rate Limiter/1 -> Multiport Switch1/2
  Multiport Switch/1 -> Terminator4/1
  Gain2/1 -> Multiport Switch1/3
  CarlaRef/1 -> Demux/1
  Demux/1 -> Gain2/1
  Demux/2 -> Terminator2/1
  Demux/3 -> Terminator3/1
  Constant/1 -> Multiport Switch1/5
  Clock1/1 -> US1/1, Add1/1
  ManSpdSel/1 -> Switch1/2, Multiport Switch1/1, Output/1
  1-D Lookup Table/1 -> Add2/1
  Add1/1 -> 1-D Lookup Table/1  "tCycle"
  SUMO Veh speed Cmd Level/1 -> Add2/2
  Switch1/1 -> Add1/2, Memory4/1
  Memory4/1 -> Switch1/1
  Gain3/1 -> Multiport Switch1/4
  Add2/1 -> Gain3/1
  Clock/1 -> Switch1/3
  US1/1 -> Rate Limiter/1

== system CAVE_MachE_Simulink_250904/Vehicle Under Test3/Vehicle/From CAN ==
  BrakeSwitch : Inport
  Brake switch ource selection : Constant  Value=2
  Bus Creator1 : BusCreator  Inputs=2
  Demux : Demux  Outputs=1
  Ground : Ground
  Ground1 : Ground
  Multiport Switch1 : MultiPortSwitch  Inputs=2  SaturateOnIntegerOverflow=off  InputSameDT=off
  IO_Out : Outport
  wires:
  Bus Creator1/1 -> IO_Out/1  "IO_Out"
  Multiport Switch1/1 -> Bus Creator1/2  "BRAKE_LAMP_BOOL_CAN"
  Demux/1 -> Bus Creator1/1  "STEERING_ANGLE_DEG_CAN"
  Ground/1 -> Demux/1
  Brake switch ource selection/1 -> Multiport Switch1/1
  Ground1/1 -> Multiport Switch1/2  "Brake switch from CAN"
  BrakeSwitch/1 -> Multiport Switch1/3

== system CAVE_MachE_Simulink_250904/Vehicle Under Test3/Vehicle/Front Wheel Drive ==
  DrvShfTrq : Inport
  Omega : Inport  Port=2
  Ideal Diff : Subsystem  VariantControl=0
  Ideal Diff AWD : Subsystem  VariantControl=Choice
  Real Diff : Subsystem  VariantControl=1
  Diff : Outport  VectorParamsAs1DForOutWhenUnconnected=off
  AxlTrq : Outport  Port=2  VectorParamsAs1DForOutWhenUnconnected=off
  PropShaftSpd : Outport  Port=3  VectorParamsAs1DForOutWhenUnconnected=off
